simulink model "MISSION"  (R2014b)
settings: Solver=ode4  StartTime=0  StopTime=11000  FixedStep=ConfParam.confOrbit.dt  RelTol=1e-3
undefined symbols (not defined in the file): ConfParam
libraries: Qinverse x2, Command x1, Date x1, Orbit x1, Estimator x1, MTBcontroller x1, RWS_PDcontroller x1, DipoleField x1, SunEphemeris_MathWorks x1, MTB x1, AeroTorqueA x1, ChangeFrame x1
settings Model: Creator=Hp  LastModifiedBy=Hp
settings DataIOCC: SaveTime=off
settings DebuggingCC: MultiTaskRateTransMsg=warning

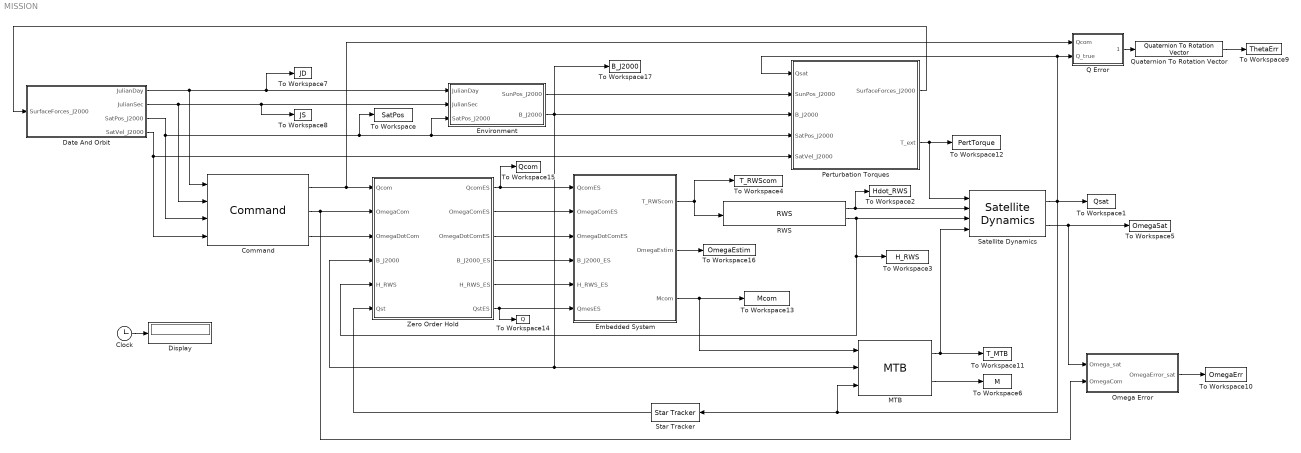
== system MISSION ==
  Clock : Clock
  Command : Command/Command
  Date And Orbit : Subsystem
  Display : Display
  Embedded System : Subsystem
  Environment : Subsystem
  MTB : MTB/MTB
  Omega Error : Subsystem
  Perturbation Torques : Subsystem
  Q Error : Subsystem
  Quaternion To Rotation Vector : Quat2Rot/Quaternion To Rotation Vector
  RWS : RWS/RWS
  Satellite Dynamics : SatDyn/Satellite Dynamics
  Star Tracker : StarTracker/Star Tracker
  To Workspace : ToWorkspace  VariableName=SatPos  SaveFormat=Timeseries  SampleTime=-1
  To Workspace1 : ToWorkspace  VariableName=Qsat  SaveFormat=Timeseries  SampleTime=-1
  To Workspace10 : ToWorkspace  VariableName=OmegaErr  SaveFormat=Timeseries  SampleTime=-1
  To Workspace11 : ToWorkspace  VariableName=T_MTB  SaveFormat=Timeseries  SampleTime=-1
  To Workspace12 : ToWorkspace  VariableName=PertTorque  SaveFormat=Timeseries  SampleTime=-1
  To Workspace13 : ToWorkspace  VariableName=Mcom  SaveFormat=Timeseries  SampleTime=-1
  To Workspace14 : ToWorkspace  VariableName=Q  SaveFormat=Timeseries  SampleTime=-1
  To Workspace15 : ToWorkspace  VariableName=Qcom  SaveFormat=Timeseries  SampleTime=-1
  To Workspace16 : ToWorkspace  VariableName=OmegaEstim  SaveFormat=Timeseries  SampleTime=-1
  To Workspace17 : ToWorkspace  VariableName=B_J2000  SaveFormat=Timeseries  SampleTime=-1
  To Workspace2 : ToWorkspace  VariableName=Hdot_RWS  SaveFormat=Timeseries  SampleTime=-1
  To Workspace3 : ToWorkspace  VariableName=H_RWS  SaveFormat=Timeseries  SampleTime=-1
  To Workspace4 : ToWorkspace  VariableName=T_RWScom  SaveFormat=Timeseries  SampleTime=-1
  To Workspace5 : ToWorkspace  VariableName=OmegaSat  SaveFormat=Timeseries  SampleTime=-1
  To Workspace6 : ToWorkspace  VariableName=M  SaveFormat=Timeseries  SampleTime=-1
  To Workspace7 : ToWorkspace  VariableName=JD  SaveFormat=Timeseries  SampleTime=-1
  To Workspace8 : ToWorkspace  VariableName=JS  SaveFormat=Timeseries  SampleTime=-1
  To Workspace9 : ToWorkspace  VariableName=ThetaErr  SaveFormat=Timeseries  SampleTime=-1
  Zero Order Hold : Subsystem
  wires:
  Command/1 -> Q Error/1(Qcom), Zero Order Hold/1(Qcom)
  Command/2 -> Omega Error/2(OmegaCom), Zero Order Hold/2(OmegaCom)
  RWS/1 -> Satellite Dynamics/2, To Workspace2/1
  MTB/1 -> Satellite Dynamics/4, To Workspace11/1
  Perturbation Torques/2(T_ext) -> To Workspace12/1, Satellite Dynamics/1
  Satellite Dynamics/2 -> To Workspace5/1, Omega Error/1(Omega_sat)
  MTB/2 -> To Workspace6/1
  Omega Error/1(OmegaError_sat) -> To Workspace10/1
  Q Error/1(Q_error) -> Quaternion To Rotation Vector/1
  Quaternion To Rotation Vector/1 -> To Workspace9/1
  Satellite Dynamics/1 -> Star Tracker/1, MTB/3, Q Error/2(Q_true), Perturbation Torques/1(Qsat), To Workspace1/1
  Environment/1(SunPos_J2000) -> Perturbation Torques/2(SunPos_J2000)
  Date And Orbit/3(SatPos_J2000) -> Command/3, To Workspace/1, Environment/3(SatPos_J2000), Perturbation Torques/4(SatPos_J2000)
  Date And Orbit/1(JulianDay) -> Command/1, Environment/1(JulianDay), To Workspace7/1
  Date And Orbit/2(JulianSec) -> Command/2, To Workspace8/1, Environment/2(JulianSec)
  Date And Orbit/4(SatVel_J2000) -> Command/4, Perturbation Torques/5(SatVel_J2000)
  Clock/1 -> Display/1
  Perturbation Torques/1(SurfaceForces_J2000) -> Date And Orbit/1(SurfaceForces_J2000)
  Embedded System/3(Mcom) -> To Workspace13/1, MTB/1
  Embedded System/1(T_RWScom) -> RWS/1, To Workspace4/1
  RWS/2 -> Satellite Dynamics/3, To Workspace3/1, Zero Order Hold/5(H_RWS)
  Zero Order Hold/6(QstES) -> To Workspace14/1, Embedded System/6(QmesES)
  Zero Order Hold/1(QcomES) -> To Workspace15/1, Embedded System/1(QcomES)
  Command/3 -> Zero Order Hold/3(OmegaDotCom)
  Star Tracker/1 -> Zero Order Hold/6(Qst)
  Zero Order Hold/2(OmegaComES) -> Embedded System/2(OmegaComES)
  Zero Order Hold/3(OmegaDotComES) -> Embedded System/3(OmegaDotComES)
  Zero Order Hold/5(H_RWS_ES) -> Embedded System/5(H_RWS_ES)
  Zero Order Hold/4(B_J2000_ES) -> Embedded System/4(B_J2000_ES)
  Embedded System/2(OmegaEstim) -> To Workspace16/1
  Environment/2(B_J2000) -> To Workspace17/1, Zero Order Hold/4(B_J2000), MTB/2, Perturbation Torques/3(B_J2000)

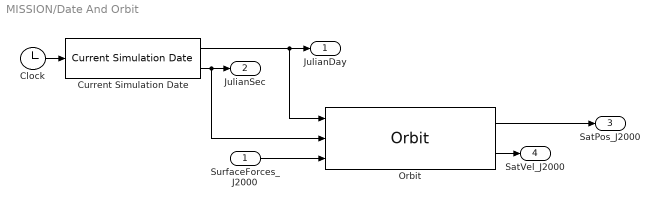
== system MISSION/Date And Orbit ==
  SurfaceForces_J2000 : Inport
  Clock : Clock
      settings: Decimation=1/ConfParam.confOrbit.dt
  Current Simulation Date : Date/Current Simulation Date
  Orbit : Orbit/Orbit
  JulianDay : Outport
  JulianSec : Outport  Port=2
  SatPos_J2000 : Outport  Port=3
  SatVel_J2000 : Outport  Port=4
  wires:
  Orbit/2 -> SatVel_J2000/1
  Clock/1 -> Current Simulation Date/1
  Current Simulation Date/1 -> Orbit/1, JulianDay/1
  Orbit/1 -> SatPos_J2000/1
  Current Simulation Date/2 -> Orbit/2, JulianSec/1
  SurfaceForces_J2000/1 -> Orbit/3

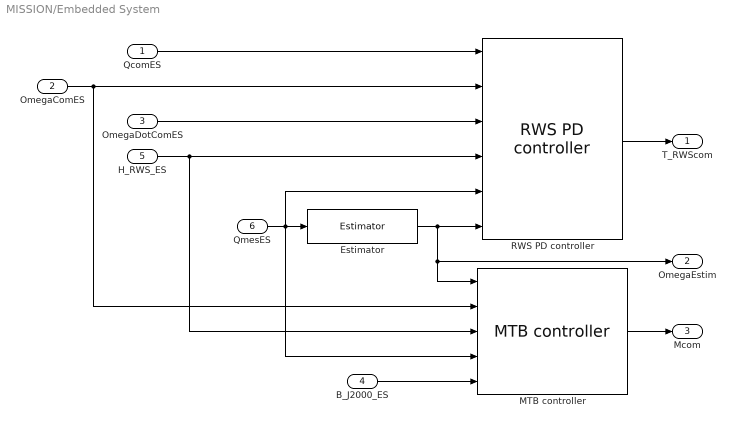
== system MISSION/Embedded System ==
  QcomES : Inport
  OmegaComES : Inport  Port=2
  OmegaDotComES : Inport  Port=3
  B_J2000_ES : Inport  Port=4
  H_RWS_ES : Inport  Port=5
  QmesES : Inport  Port=6
  Estimator : Estimator/Estimator
  MTB controller : MTBcontroller/MTB controller
  RWS PD controller : RWS_PDcontroller/RWS PD controller
  T_RWScom : Outport
  OmegaEstim : Outport  Port=2
  Mcom : Outport  Port=3
  wires:
  QmesES/1 -> Estimator/1, RWS PD controller/5, MTB controller/4
  QcomES/1 -> RWS PD controller/1
  RWS PD controller/1 -> T_RWScom/1
  Estimator/1 -> RWS PD controller/6, MTB controller/1, OmegaEstim/1
  H_RWS_ES/1 -> MTB controller/3, RWS PD controller/4
  B_J2000_ES/1 -> MTB controller/5
  OmegaComES/1 -> MTB controller/2, RWS PD controller/2
  OmegaDotComES/1 -> RWS PD controller/3
  MTB controller/1 -> Mcom/1

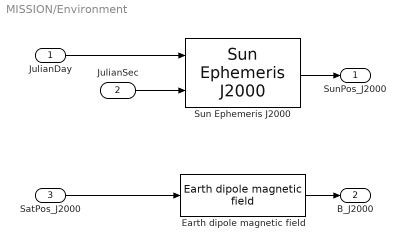
== system MISSION/Environment ==
  JulianDay : Inport
  JulianSec : Inport  Port=2
  SatPos_J2000 : Inport  Port=3
  Earth dipole magnetic field : DipoleField/Earth dipole magnetic field
  Sun Ephemeris J2000 : SunEphemeris_MathWorks/Sun Ephemeris J2000
  SunPos_J2000 : Outport
  B_J2000 : Outport  Port=2
  wires:
  Sun Ephemeris J2000/1 -> SunPos_J2000/1
  JulianSec/1 -> Sun Ephemeris J2000/2
  SatPos_J2000/1 -> Earth dipole magnetic field/1
  JulianDay/1 -> Sun Ephemeris J2000/1
  Earth dipole magnetic field/1 -> B_J2000/1

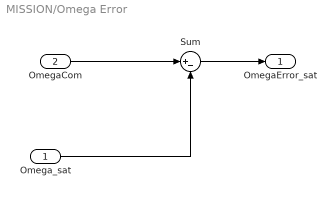
== system MISSION/Omega Error ==
  Omega_sat : Inport
  OmegaCom : Inport  Port=2
  Sum : Sum  Inputs=|+-
  OmegaError_sat : Outport
  wires:
  Omega_sat/1 -> Sum/2
  OmegaCom/1 -> Sum/1
  Sum/1 -> OmegaError_sat/1

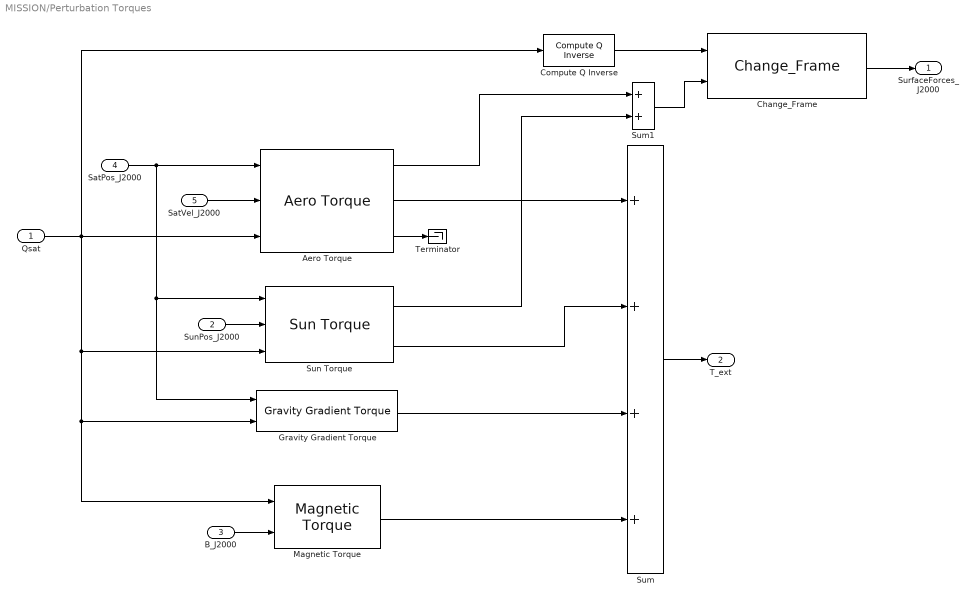
== system MISSION/Perturbation Torques ==
  Qsat : Inport
  SunPos_J2000 : Inport  Port=2
  B_J2000 : Inport  Port=3
  SatPos_J2000 : Inport  Port=4
  SatVel_J2000 : Inport  Port=5
  Aero Torque : AeroTorqueA/Aero Torque
  Change_Frame : ChangeFrame/Change_Frame
  Compute Q Inverse : Qinverse/Compute Q Inverse
  Gravity Gradient Torque : GravGradTorque/Gravity Gradient Torque
  Magnetic Torque : MagnTorque/Magnetic Torque
  Sum : Sum  Inputs=++++
  Sum1 : Sum
  Sun Torque : SunTorqueA/Sun Torque
  Terminator : Terminator
  SurfaceForces_J2000 : Outport
  T_ext : Outport  Port=2
  wires:
  SunPos_J2000/1 -> Sun Torque/2
  SatVel_J2000/1 -> Aero Torque/2
  Qsat/1 -> Compute Q Inverse/1, Magnetic Torque/1, Gravity Gradient Torque/2, Sun Torque/3, Aero Torque/3
  Gravity Gradient Torque/1 -> Sum/3
  Sun Torque/1 -> Sum1/2
  Aero Torque/3 -> Terminator/1
  B_J2000/1 -> Magnetic Torque/2
  Sum/1 -> T_ext/1
  Magnetic Torque/1 -> Sum/4
  Sun Torque/2 -> Sum/2
  SatPos_J2000/1 -> Aero Torque/1, Gravity Gradient Torque/1, Sun Torque/1
  Compute Q Inverse/1 -> Change_Frame/1
  Sum1/1 -> Change_Frame/2
  Change_Frame/1 -> SurfaceForces_J2000/1
  Aero Torque/1 -> Sum1/1
  Aero Torque/2 -> Sum/1

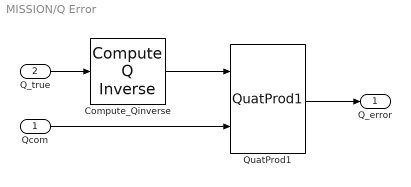
== system MISSION/Q Error ==
  Qcom : Inport
  Q_true : Inport  Port=2
  Compute_Qinverse : Qinverse/Compute Q Inverse
  QuatProd1 : Qprod/QuatProd1
  Q_error : Outport
  wires:
  QuatProd1/1 -> Q_error/1
  Qcom/1 -> QuatProd1/2
  Compute_Qinverse/1 -> QuatProd1/1
  Q_true/1 -> Compute_Qinverse/1

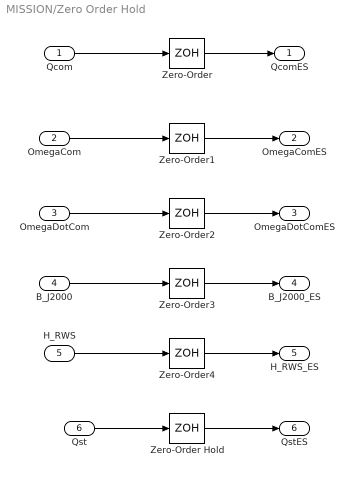
== system MISSION/Zero Order Hold ==
  Qcom : Inport
  OmegaCom : Inport  Port=2
  OmegaDotCom : Inport  Port=3
  B_J2000 : Inport  Port=4
  H_RWS : Inport  Port=5
  Qst : Inport  Port=6
  Zero-Order{,1..4} (5 alike) : ZeroOrderHold  SampleTime=1/ConfParam.confES.frequency
  Zero-Order Hold : ZeroOrderHold  SampleTime=1/ConfParam.confES.frequency
  QcomES : Outport
  OmegaComES : Outport  Port=2
  OmegaDotComES : Outport  Port=3
  B_J2000_ES : Outport  Port=4
  H_RWS_ES : Outport  Port=5
  QstES : Outport  Port=6
  wires:
  Qst/1 -> Zero-Order Hold/1
  Zero-Order4/1 -> H_RWS_ES/1
  Qcom/1 -> Zero-Order/1
  H_RWS/1 -> Zero-Order4/1
  OmegaCom/1 -> Zero-Order1/1
  B_J2000/1 -> Zero-Order3/1
  OmegaDotCom/1 -> Zero-Order2/1
  Zero-Order1/1 -> OmegaComES/1
  Zero-Order2/1 -> OmegaDotComES/1
  Zero-Order3/1 -> B_J2000_ES/1
  Zero-Order/1 -> QcomES/1
  Zero-Order Hold/1 -> QstES/1
